simulink model "fuzzy_control"  (R2020b)
settings: Solver=FixedStepAuto  StartTime=0.0  StopTime=20  FixedStep=0.009  RelTol=1e-3
undefined symbols (not defined in the file or in its folder): magnitude
libraries: simulink x2, simulink_extras x1, fuzblock x1
settings Model: PauseTimes=2.78  Creator=alvar  LastModifiedBy=juanj

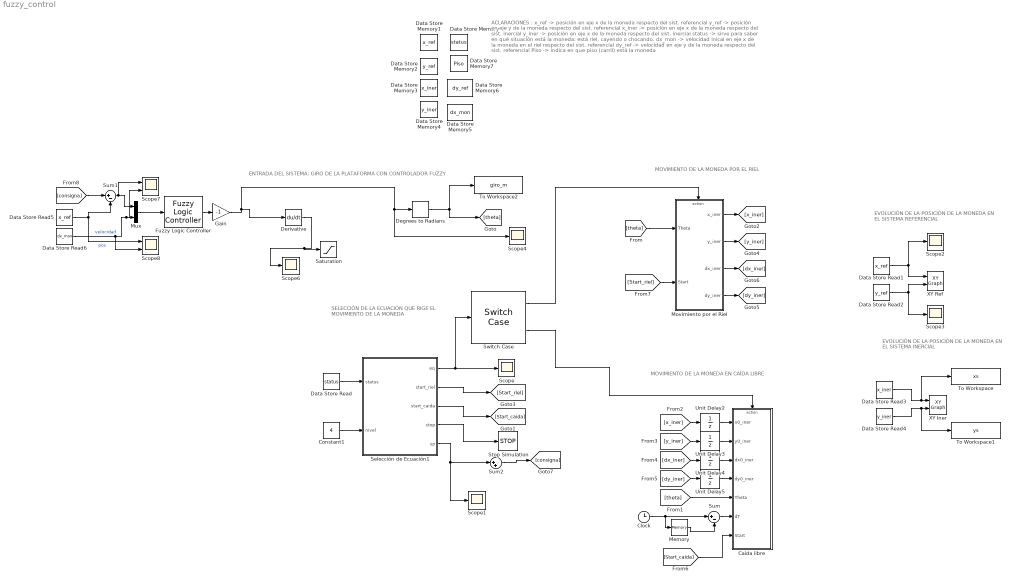
== system fuzzy_control ==
  note: ENTRADA DEL SISTEMA: GIRO DE LA PLATAFORMA CON CONTROLADOR FUZZY
  note: SELECCIÓN DE LA ECUACIÓN QUE RIGE EL MOVIMIENTO DE LA MONEDA
  note: MOVIMIENTO DE LA MONEDA EN CAÍDA LIBRE
  note: MOVIMIENTO DE LA MONEDA POR EL RIEL
  note: EVOLUCIÓN DE LA POSICIÓN DE LA MONEDA EN EL SISTEMA REFERENCIAL
  note: ACLARACIONES :
      |
      | x_ref -> posición en eje x de la moneda respecto del sist. referencial
      | y_ref -> posición en eje y de la moneda respecto del sist. referencial
      |
      | x_iner -> posición en eje x de la moneda respecto del sist. inercial
      | y_iner -> posición en eje x de la moneda respecto del sist. inercial
      |
      | status -> sirve para saber en qué situación está la moneda: está riel, cayendo o chocando.
      |
      | dx_mon -> velocidad inical en eje x de la moneda en el riel respecto del sist. referencial
      |
      | dy_ref -> velocidad en eje y de la moneda respecto del sist. referencial
      |
      | Piso -> indica en que piso (carril) está la moneda
  note: EVOLUCIÓN DE LA POSICIÓN DE LA MONEDA EN EL SISTEMA INERCIAL
  Caida libre : Subsystem  TreatAsAtomicUnit=on
  Clock : Clock
  Constant1 : Constant  Value=4
  Data Store Memory : DataStoreMemory  DataStoreName=status  ReadBeforeWriteMsg=warning  WriteAfterWriteMsg=warning  WriteAfterReadMsg=warning  ShowAdditionalParam=off  OutDataTypeStr=double
  Data Store Memory1 : DataStoreMemory  DataStoreName=x_ref  ReadBeforeWriteMsg=warning  WriteAfterWriteMsg=warning  WriteAfterReadMsg=warning  InitialValue=-0.11  ShowAdditionalParam=off  OutDataTypeStr=double
  Data Store Memory2 : DataStoreMemory  DataStoreName=y_ref  ReadBeforeWriteMsg=warning  WriteAfterWriteMsg=warning  WriteAfterReadMsg=warning  ShowAdditionalParam=off  OutDataTypeStr=double
  Data Store Memory3 : DataStoreMemory  DataStoreName=x_iner  ReadBeforeWriteMsg=warning  WriteAfterWriteMsg=warning  WriteAfterReadMsg=warning  InitialValue=-0.11  ShowAdditionalParam=off  OutDataTypeStr=double
  Data Store Memory4 : DataStoreMemory  DataStoreName=y_iner  ReadBeforeWriteMsg=warning  WriteAfterWriteMsg=warning  WriteAfterReadMsg=warning  ShowAdditionalParam=off  OutDataTypeStr=double
  Data Store Memory5 : DataStoreMemory  DataStoreName=dx_mon  ReadBeforeWriteMsg=warning  WriteAfterWriteMsg=warning  WriteAfterReadMsg=warning  ShowAdditionalParam=off  OutDataTypeStr=double
  Data Store Memory6 : DataStoreMemory  DataStoreName=dy_ref  ReadBeforeWriteMsg=warning  WriteAfterWriteMsg=warning  WriteAfterReadMsg=warning  ShowAdditionalParam=off  OutDataTypeStr=double
  Data Store Memory7 : DataStoreMemory  DataStoreName=Piso  ReadBeforeWriteMsg=warning  WriteAfterWriteMsg=warning  WriteAfterReadMsg=warning  InitialValue=1  ShowAdditionalParam=off  OutDataTypeStr=double
  Data Store Read : DataStoreRead  DataStoreName=status
  Data Store Read1 : DataStoreRead  DataStoreName=x_ref
  Data Store Read2 : DataStoreRead  DataStoreName=y_ref
  Data Store Read3 : DataStoreRead  DataStoreName=x_iner
  Data Store Read4 : DataStoreRead  DataStoreName=y_iner
  Data Store Read5 : DataStoreRead  DataStoreName=x_ref
  Data Store Read6 : DataStoreRead  DataStoreName=dx_mon
  Degrees to Radians : simulink_extras/Transformations/Degrees to Radians
  Derivative : Derivative
  Fuzzy Logic Controller : fuzblock/Fuzzy Logic  Controller  FIS='fuzzy_controller4.fis'  OutputSampleNumber=101  DataType=double  FuzzifiedInputs=off  RuleFiringStrengths=off  RuleOutputs=off  AggregatedOutputs=off  SimulateUsing=Interpreted execution  OutOfRangeInputValueMessage=warning  NoRuleFiredMessage=warning  EmptyOutputFuzzySetMessage=warning
  Gain : Gain  Gain=-1
  Memory : Memory
  Movimiento por el Riel : Subsystem  TreatAsAtomicUnit=on
  Mux : Mux  Inputs=2
  Saturation : Saturate  UpperLimit=300  LowerLimit=-300
  Scope{,1..4,6} (6 alike) : Scope
  Scope7 : Scope  NumInputPorts=2
  Scope8 : Scope  NumInputPorts=2
  Selección de Ecuación1 : MATLAB Function  TreatAsAtomicUnit=on
  Stop Simulation : Stop
  Sum : Sum  Inputs=|+-
  Sum1 : Sum  Inputs=|+-
  Sum2 : Sum  Inputs=|++
  Switch Case : SwitchCase  CaseConditions={1,2}  ShowDefaultCase=off
  To Workspace : ToWorkspace  VariableName=xs  SampleTime=-1
  To Workspace1 : ToWorkspace  VariableName=ys  SampleTime=-1
  To Workspace2 : ToWorkspace  VariableName=giro_m  SampleTime=-1
  Unit Delay{2..5} (4 alike) : UnitDelay  SampleTime=-1  HasFrameUpgradeWarning=on
  XY Iner : simulink/Sinks/XY Graph  xmin=-0.15  xmax=0.15  ymin=-0.3  ymax=0.2  st=-1
  XY Ref : simulink/Sinks/XY Graph  xmin=-0.2  xmax=0.2  ymin=-0.3  ymax=0.2  st=-1
  wires:
  Switch Case/1 -> Movimiento por el Riel/Action
  [theta] -> Movimiento por el Riel/1(Theta)
  Switch Case/2 -> Caida libre/Action
  Selección de Ecuación1/1(eq) -> Scope/1, Switch Case/1
  Data Store Read/1 -> Selección de Ecuación1/1(status)
  Degrees to Radians/1 -> To Workspace2/1, [theta]
  Memory/1 -> Sum/2
  Clock/1 -> Sum/1, Memory/1
  Sum/1 -> Caida libre/6(dT)
  [x_iner] -> Unit Delay2/1
  Unit Delay2/1 -> Caida libre/1(x0_iner)
  [y_iner] -> Unit Delay3/1
  Unit Delay3/1 -> Caida libre/2(y0_iner)
  [dx_iner] -> Unit Delay4/1
  Unit Delay4/1 -> Caida libre/3(dx0_iner)
  [dy_iner] -> Unit Delay5/1
  Unit Delay5/1 -> Caida libre/4(dy0_iner)
  [theta] -> Caida libre/5(Theta)
  Data Store Read1/1 -> Scope2/1, XY Ref/1
  Data Store Read2/1 -> Scope3/1, XY Ref/2
  Data Store Read4/1 -> To Workspace1/1, XY Iner/2
  Data Store Read3/1 -> To Workspace/1, XY Iner/1
  Movimiento por el Riel/1(x_iner) -> [x_iner]
  Movimiento por el Riel/3(dx_iner) -> [dx_iner]
  Movimiento por el Riel/2(y_iner) -> [y_iner]
  Movimiento por el Riel/4(dy_iner) -> [dy_iner]
  Selección de Ecuación1/3(start_caida) -> [Start_caida]
  [Start_caida] -> Caida libre/7(Start)
  Constant1/1 -> Selección de Ecuación1/2(nivel)
  Selección de Ecuación1/4(stop) -> Stop Simulation/1
  Selección de Ecuación1/2(start_riel) -> [Start_riel]
  [Start_riel] -> Movimiento por el Riel/2(Start)
  Fuzzy Logic Controller/1 -> Gain/1
  Data Store Read5/1 -> Sum1/2, Scope8/1  "pos"
  Selección de Ecuación1/5(sp) -> Sum2/1, Scope1/1
  Mux/1 -> Fuzzy Logic Controller/1
  Sum1/1 -> Scope7/1, Mux/1
  Data Store Read6/1 -> Scope8/2, Scope7/2, Mux/2  "velocidad"
  [consigna] -> Sum1/1
  Sum2/1 -> [consigna]
  Derivative/1 -> Saturation/1, Scope6/1
  Gain/1 -> Scope4/1, Degrees to Radians/1, Derivative/1

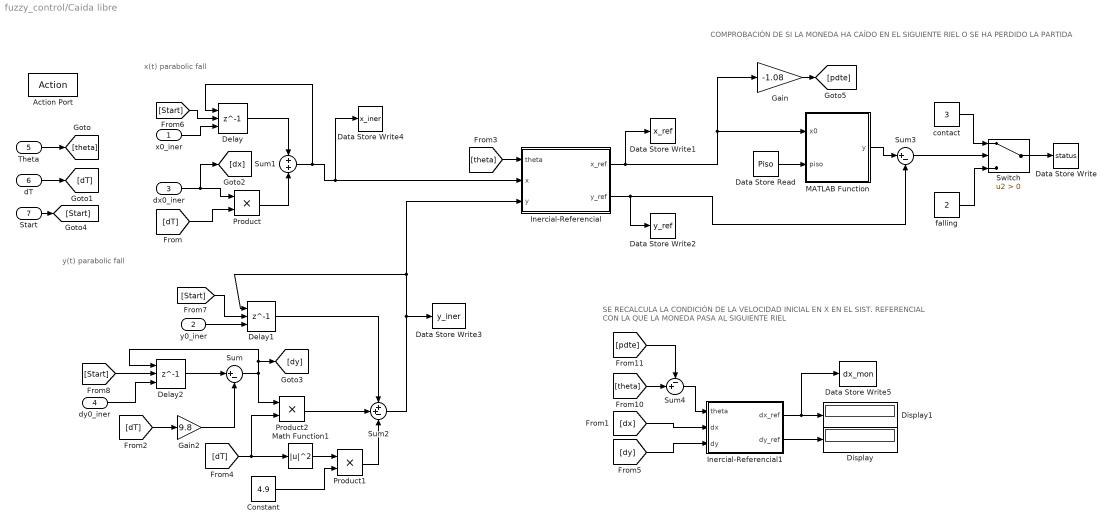
== system fuzzy_control/Caida libre ==
  note: SE RECALCULA LA CONDICIÓN DE LA VELOCIDAD INICIAL EN X EN EL SIST. REFERENCIAL CON LA QUE LA MONEDA PASA AL SIGUIENTE RIEL
  note: COMPROBACIÓN DE SI LA MONEDA HA CAÍDO EN EL SIGUIENTE RIEL O SE HA PERDIDO LA PARTIDA
  note: x(t) parabolic fall
  note: y(t) parabolic fall
  x0_iner : Inport
  y0_iner : Inport  Port=2
  dx0_iner : Inport  Port=3
  dy0_iner : Inport  Port=4
  Theta : Inport  Port=5
  dT : Inport  Port=6
  Start : Inport  Port=7
  Action Port : ActionPort  ActionPortLabel=case [ 2 ]:
  Constant : Constant  Value=4.9
  Data Store Read : DataStoreRead  DataStoreName=Piso
  Data Store Write : DataStoreWrite  DataStoreName=status
  Data Store Write1 : DataStoreWrite  DataStoreName=x_ref
  Data Store Write2 : DataStoreWrite  DataStoreName=y_ref
  Data Store Write3 : DataStoreWrite  DataStoreName=y_iner
  Data Store Write4 : DataStoreWrite  DataStoreName=x_iner
  Data Store Write5 : DataStoreWrite  DataStoreName=dx_mon
  Delay : Delay  DelayLength=1  InitialConditionSource=Input port  ExternalReset=Rising
      settings: InputPortMap=u0,r5,p4
  Delay1 : Delay  DelayLength=1  InitialConditionSource=Input port  ExternalReset=Rising
      settings: InputPortMap=u0,r5,p4
  Delay2 : Delay  DelayLength=1  InitialConditionSource=Input port  ExternalReset=Rising
      settings: InputPortMap=u0,r5,p4
  Display : Display
  Display1 : Display
  Gain : Gain  Gain=-1.08
  Gain2 : Gain  Gain=9.8
  Inercial-Referencial : MATLAB Function  TreatAsAtomicUnit=on
  Inercial-Referencial1 : MATLAB Function  TreatAsAtomicUnit=on
  MATLAB Function : MATLAB Function  TreatAsAtomicUnit=on
  Math Function1 : Math  Operator=magnitude^2  SaturateOnIntegerOverflow=on
  Product : Product
  Product1 : Product
  Product2 : Product
  Sum : Sum  Inputs=|+-
  Sum1 : Sum
  Sum2 : Sum  Inputs=++-
  Sum3 : Sum  Inputs=|+-
  Sum4 : Sum  Inputs=-+|
  Switch : Switch  Criteria=u2 > Threshold
  contact : Constant  Value=3
  falling : Constant  Value=2
  wires:
  [dT] -> Product/2
  Product/1 -> Sum1/2
  Delay1/1 -> Sum2/1
  [dT] -> Product2/2, Math Function1/1
  Sum1/1 -> Data Store Write4/1, Inercial-Referencial/2(x), Delay/1
  Product2/1 -> Sum2/2
  Product1/1 -> Sum2/3
  Math Function1/1 -> Product1/1
  Theta/1 -> [theta]
  x0_iner/1 -> Delay/3
  Delay/1 -> Sum1/1
  dT/1 -> [dT]
  dx0_iner/1 -> Product/1, [dx]
  y0_iner/1 -> Delay1/3
  Sum2/1 -> Inercial-Referencial/3(y), Delay1/1, Data Store Write3/1
  dy0_iner/1 -> Delay2/3
  Delay2/1 -> Sum/1
  [dT] -> Gain2/1
  Gain2/1 -> Sum/2
  Sum/1 -> Product2/1, [dy], Delay2/1
  [theta] -> Inercial-Referencial/1(theta)
  Constant/1 -> Product1/2
  [dx] -> Inercial-Referencial1/2(dx)
  [dy] -> Inercial-Referencial1/3(dy)
  Inercial-Referencial/1(x_ref) -> Gain/1, MATLAB Function/1(x0), Data Store Write1/1
  Data Store Read/1 -> MATLAB Function/2(piso)
  MATLAB Function/1(y) -> Sum3/1
  Inercial-Referencial/2(y_ref) -> Sum3/2, Data Store Write2/1
  falling/1 -> Switch/3
  Sum3/1 -> Switch/2
  Switch/1 -> Data Store Write/1
  contact/1 -> Switch/1
  Inercial-Referencial1/1(dx_ref) -> Data Store Write5/1, Display1/1
  Inercial-Referencial1/2(dy_ref) -> Display/1
  Start/1 -> [Start]
  [Start] -> Delay/2
  [Start] -> Delay1/2
  [Start] -> Delay2/2
  Gain/1 -> [pdte]
  [theta] -> Sum4/2
  [pdte] -> Sum4/1
  Sum4/1 -> Inercial-Referencial1/1(theta)

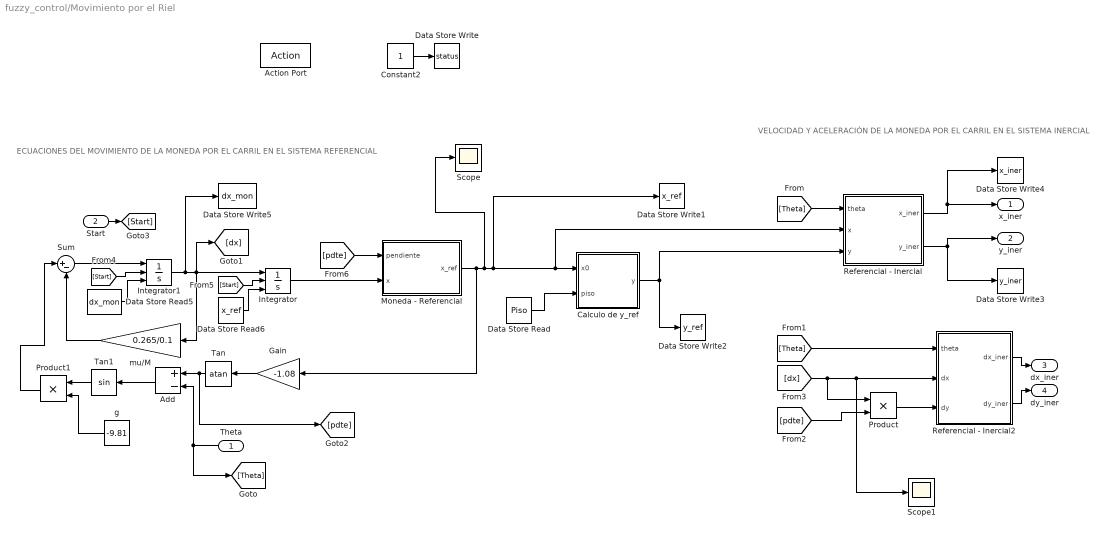
== system fuzzy_control/Movimiento por el Riel ==
  note: VELOCIDAD Y ACELERACIÓN DE LA MONEDA POR EL CARRIL EN EL SISTEMA INERCIAL
  note: ECUACIONES DEL MOVIMIENTO DE LA MONEDA POR EL CARRIL EN EL SISTEMA REFERENCIAL
  Theta : Inport
  Start : Inport  Port=2
  Action Port : ActionPort  ActionPortLabel=case [ 1 ]:
  Add : Sum  Inputs=+-
  Calculo de y_ref : MATLAB Function  TreatAsAtomicUnit=on
  Constant2 : Constant
  Data Store Read : DataStoreRead  DataStoreName=Piso
  Data Store Read5 : DataStoreRead  DataStoreName=dx_mon
  Data Store Read6 : DataStoreRead  DataStoreName=x_ref
  Data Store Write : DataStoreWrite  DataStoreName=status
  Data Store Write1 : DataStoreWrite  DataStoreName=x_ref
  Data Store Write2 : DataStoreWrite  DataStoreName=y_ref
  Data Store Write3 : DataStoreWrite  DataStoreName=y_iner
  Data Store Write4 : DataStoreWrite  DataStoreName=x_iner
  Data Store Write5 : DataStoreWrite  DataStoreName=dx_mon
  Gain : Gain  Gain=-1.08
  Integrator : Integrator  ExternalReset=rising  InitialConditionSource=external
  Integrator1 : Integrator  ExternalReset=rising  InitialConditionSource=external
  Moneda - Referencial : MATLAB Function  TreatAsAtomicUnit=on
  Product : Product
  Product1 : Product
  Referencial - Inercial : MATLAB Function  TreatAsAtomicUnit=on
  Referencial - Inercial2 : MATLAB Function  TreatAsAtomicUnit=on
  Scope : Scope
  Scope1 : Scope
  Sum : Sum  Inputs=|+-
  Tan : Trigonometry  Operator=atan
  Tan1 : Trigonometry
  g : Constant  Value=-9.81
  mu/M : Gain  Gain=0.265/0.1
  x_iner : Outport
  y_iner : Outport  Port=2
  dx_iner : Outport  Port=3
  dy_iner : Outport  Port=4
  wires:
  Add/1 -> Tan1/1
  Tan/1 -> [pdte], Add/1
  Gain/1 -> Tan/1
  mu/M/1 -> Sum/2
  g/1 -> Product1/2
  Integrator1/1 -> Data Store Write5/1, [dx], mu/M/1, Integrator/1
  Data Store Read5/1 -> Integrator1/3
  Sum/1 -> Integrator1/1
  Tan1/1 -> Product1/1
  Data Store Read6/1 -> Integrator/3
  Theta/1 -> [Theta], Add/2
  Data Store Read/1 -> Calculo de y_ref/2(piso)
  Calculo de y_ref/1(y) -> Referencial - Inercial/3(y), Data Store Write2/1
  Constant2/1 -> Data Store Write/1
  Referencial - Inercial/1(x_iner) -> Data Store Write4/1, x_iner/1
  Referencial - Inercial/2(y_iner) -> Data Store Write3/1, y_iner/1
  [Theta] -> Referencial - Inercial/1(theta)
  [Theta] -> Referencial - Inercial2/1(theta)
  Referencial - Inercial2/2(dy_iner) -> dy_iner/1
  Referencial - Inercial2/1(dx_iner) -> dx_iner/1
  [dx] -> Scope1/1, Referencial - Inercial2/2(dx), Product/1
  Product/1 -> Referencial - Inercial2/3(dy)
  [pdte] -> Product/2
  Start/1 -> [Start]
  [Start] -> Integrator1/2
  [Start] -> Integrator/2
  Integrator/1 -> Moneda - Referencial/2(x)
  Moneda - Referencial/1(x_ref) -> Calculo de y_ref/1(x0), Referencial - Inercial/2(x), Data Store Write1/1, Scope/1, Gain/1
  [pdte] -> Moneda - Referencial/1(pendiente)
  Product1/1 -> Sum/1

== matlab function fuzzy_control/Movimiento por el Riel/Moneda - Referencial ==
  settings: updateMethod=DISCRETE
  data: pendiente input; x_ref output; x input
function x_ref  = rotate(pendiente,x)
x_ref =  x*cos(-pendiente);

== matlab function fuzzy_control/Movimiento por el Riel/Calculo de y_ref ==
  data: x0 input; y output; piso input
function y  = fcn(x0, piso)

switch piso
    case 1
        y= -0.54*x0^2 + 0.1143;
    case 2
        y= -0.54*x0^2 + 0.0686;
    case 3
        y= -0.54*x0^2 + 0.03;
    case 4
        y= -0.54*x0^2 - 0.03;  
    case 5
        y= -0.54*x0^2 - 0.0686; 
    case 6
        y= -0.54*x0^2 - 0.1143;
    case 7
        y= -0.54*x0^2 - 0.16;
    otherwise
        y = 0;
end

== matlab function fuzzy_control/Caida libre/Inercial-Referencial ==
  settings: updateMethod=DISCRETE
  data: theta input; x_ref output; x input; y input; y_ref output
function [x_ref,y_ref] = rotate(theta,x,y)
x_ref = x*cos(theta) - y*sin(theta);
y_ref = x*sin(theta) + y*cos(theta);

== matlab function fuzzy_control/Caida libre/Inercial-Referencial1 ==
  settings: updateMethod=DISCRETE
  data: theta input; dx_ref output; dx input; dy input; dy_ref output
function [dx_ref,dy_ref] = rotate(theta,dx,dy)
dx_ref = dx*cos(theta) - dy*sin(theta);
dy_ref = dx*sin(theta) + dy*cos(theta);

== matlab function fuzzy_control/Selección de Ecuación1 ==
  settings: updateMethod=DISCRETE
  data: eq output; status input; x_ref data_store_memory; Piso data_store_memory; start_riel output; start_caida output; stop output; nivel input; sp output
function [eq, start_riel, start_caida, stop, sp] = fcn(status, nivel)

%%DE MOMENTO ESTE CÓDIGO ES PARA PROBAR LAS ECUACIONES EN LA PRIMERA CAIDA
persistent x_edges
persistent equation
global x_ref;
global Piso;
start_riel = 0;
start_caida = 0;
stop = 0;
sp=0;
if(isempty(equation))
    equation = 1;
end
coder.extrinsic('fallCoor');
if (isempty(x_edges))
    x_edges = zeros(7,2);
    x_edges = fallCoor(nivel);
end
%x_edges = fallCoor(1)

if(status == 1)
    switch Piso
        case 1
            sp=x_edges(1,1);
            if (x_ref > x_edges(1,1)) % empieza a caer
              equation = 2; % se utiliza las ecuaciones de caída libre
              start_caida = 1; % se resetean los bloques delay
            elseif (x_ref < x_edges(1,2))
                stop = 1;
            end
            
        case 2
            sp=x_edges(2,2);
            if (x_ref < x_edges(2,2))
                equation = 2;
                start_caida = 1;
            elseif (x_ref > x_edges(2,1))
                stop = 1;
                disp('Caida Piso1');
            end
        case 3
            sp=x_edges(3,1);
            if (x_ref > x_edges(3,1))
                equation = 2;
                start_caida = 1;
            elseif (x_ref < x_edges(3,2))
                stop = 1;
            end
        case 4
            sp=x_edges(4,2);
            if (x_ref < x_edges(4,2))
                equation = 2;
                start_caida = 1;
            elseif (x_ref > x_edges(4,1))
                stop = 1;
            end
        case 5
            sp=x_edges(5,1);
            if (x_ref > x_edges(5,1))
                equation = 2;
                start_caida = 1;
            elseif (x_ref < x_edges(5,2))
                stop = 1;
            end
        case 6
            sp=x_edges(6,2);
            if (x_ref < x_edges(6,2))
                equation = 2;
                start_caida = 1;
            elseif (x_ref > x_edges(6,1))
                stop = 1;
            end
        case 7
            sp=x_edges(7,1)+0.005;
            if (x_ref > x_edges(7,1))
                equation = 2;
                start_caida = 1;
            elseif (x_ref < x_edges(7,2))
                stop = 1;
            end
    end
end

if(status == 3) % impacto
    equation = 1; % se utiliza el bloque movimiento por el riel
    Piso = Piso + 1; % se pasa al siguiente piso
    start_riel = 1; % se reseta el integrador 
end

eq = equation;

== matlab function fuzzy_control/Caida libre/MATLAB Function ==
  data: x0 input; y output; piso input
function y  = fcn(x0, piso)

paux = piso+1;
switch paux
    case 1
        y= -0.54*x0^2 + 0.1143;
    case 2
        y= -0.54*x0^2 + 0.0686;
    case 3
        y= -0.54*x0^2 + 0.03;
    case 4
        y= -0.54*x0^2 - 0.03;
    case 5
        y= -0.54*x0^2 - 0.0686; 
    case 6
        y= -0.54*x0^2 - 0.1143;
    case 7
        y= -0.54*x0^2 - 0.16;
    otherwise
        y = 0;
end

== matlab function fuzzy_control/Movimiento por el Riel/Referencial - Inercial ==
  settings: updateMethod=DISCRETE
  data: theta input; x_iner output; x input; y input; y_iner output
function [x_iner,y_iner] = rotate(theta,x,y)
x_iner =  x*cos(theta) + y*sin(theta);
y_iner = -x*sin(theta) + y*cos(theta);

== matlab function fuzzy_control/Movimiento por el Riel/Referencial - Inercial2 ==
  settings: updateMethod=DISCRETE
  data: theta input; dx_iner output; dx input; dy input; dy_iner output
function [dx_iner,dy_iner] = rotate(theta,dx,dy)
dx_iner =  dx*cos(-theta) - dy*sin(-theta);
dy_iner = dx*sin(-theta) + dy*cos(-theta);
